simulink model "h2t_TestBed"  (R2015a)
settings: Solver=FixedStepDiscrete  StartTime=0.0  StopTime=1  FixedStep=1  RelTol=1e-3
undefined symbols (not defined in the file): MWS
libraries: Lib_Thermo_Enth2Temp_TMATS x1
settings Model: Creator=jwchapm2  LastModifiedBy=jwchapm2
settings OptimizationCC: ExpressionDepthLimit=2147483647
settings DebuggingCC: UnderspecifiedInitializationDetection=Classic  MergeDetectMultiDrivingBlocksExec=none  SolverPrmCheckMsg=warning  StateNameClashWarn=warning

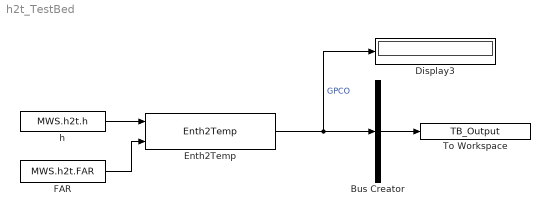
== system h2t_TestBed ==
  Bus Creator : BusCreator  Inputs=1
  Display3 : Display
  Enth2Temp : Lib_Thermo_Enth2Temp_TMATS/Enth2Temp
  FAR : Constant  Value=MWS.h2t.FAR
  To Workspace : ToWorkspace  VariableName=TB_Output  SampleTime=-1
  h : Constant  Value=MWS.h2t.h
  wires:
  FAR/1 -> Enth2Temp/2
  h/1 -> Enth2Temp/1
  Enth2Temp/1 -> Display3/1, Bus Creator/1  "GPCO"
  Bus Creator/1 -> To Workspace/1
